simulink model "sim_req"  (R2021b)
settings: Solver=VariableStepAuto  StartTime=0.0  StopTime=10.0  RelTol=1e-3
settings Model: Creator=matas  LastModifiedBy=matas

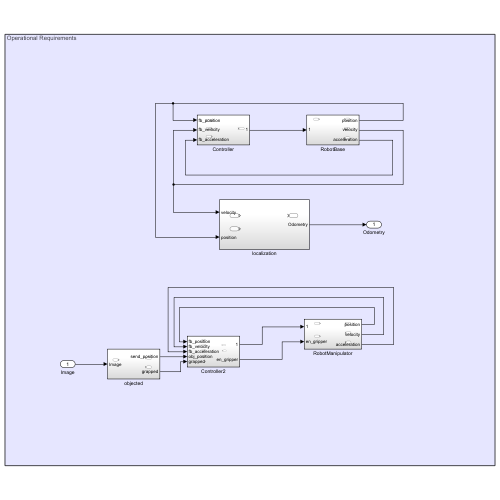
[thumbnail: Simulink's stored preview of the top-level diagram]
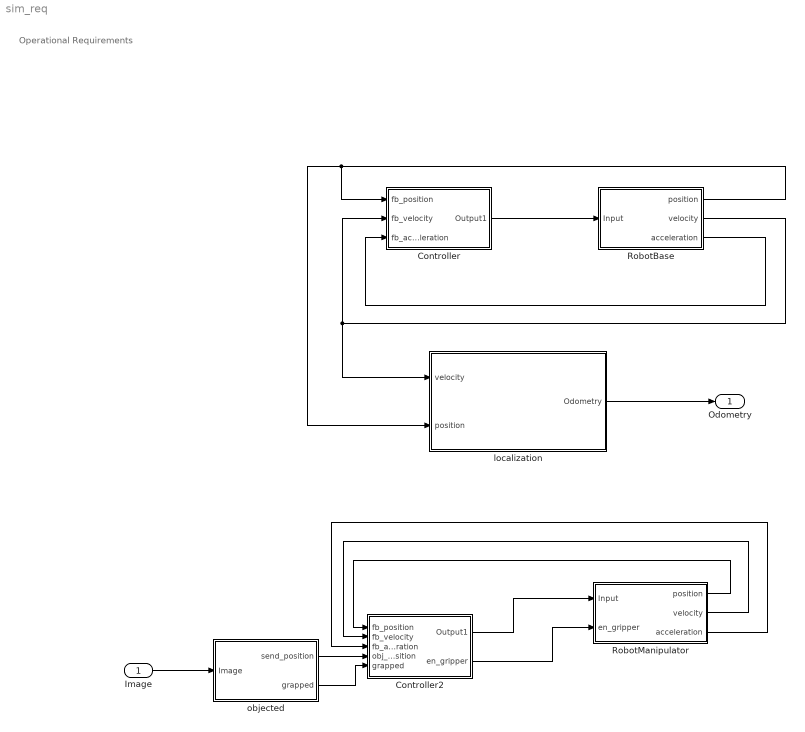
== system sim_req ==
  note: Operational Requirements
  Image : Inport
  Controller : Subsystem
  Controller2 : Subsystem
  RobotBase : Subsystem
  RobotManipulator : Subsystem
  localization : Subsystem
  objected : Subsystem
  Odometry : Outport
  wires:
  Controller/1(Output1) -> RobotBase/1(Input)
  RobotBase/1(position) -> Controller/1(fb_position), localization/2("position ")
  RobotBase/2(velocity) -> Controller/2(fb_velocity), localization/1(velocity)
  RobotBase/3(acceleration) -> Controller/3(fb_acceleration)
  localization/1(Odometry) -> Odometry/1
  RobotManipulator/1(position) -> Controller2/1(fb_position)
  RobotManipulator/2(velocity) -> Controller2/2(fb_velocity)
  RobotManipulator/3(acceleration) -> Controller2/3(fb_acceleration)
  Controller2/1(Output1) -> RobotManipulator/1(Input)
  Image/1 -> objected/1(Image)
  objected/1(send_position) -> Controller2/4(obj_position)
  Controller2/2(en_gripper) -> RobotManipulator/2(en_gripper)
  objected/2(grapped) -> Controller2/5(grapped)

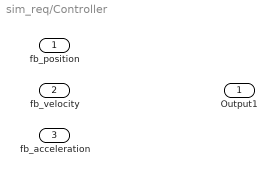
== system sim_req/Controller ==
  fb_position : Inport
  fb_velocity : Inport  Port=2
  fb_acceleration : Inport  Port=3
  Output1 : Outport

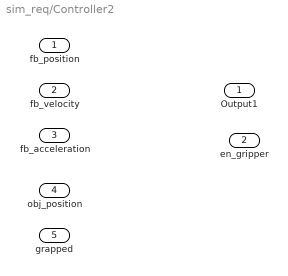
== system sim_req/Controller2 ==
  fb_position : Inport
  fb_velocity : Inport  Port=2
  fb_acceleration : Inport  Port=3
  obj_position : Inport  Port=4
  grapped : Inport  Port=5
  Output1 : Outport
  en_gripper : Outport  Port=2

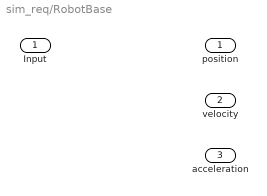
== system sim_req/RobotBase ==
  Input : Inport
  position : Outport
  velocity : Outport  Port=2
  acceleration : Outport  Port=3

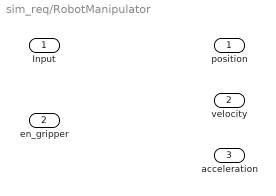
== system sim_req/RobotManipulator ==
  Input : Inport
  en_gripper : Inport  Port=2
  position : Outport
  velocity : Outport  Port=2
  acceleration : Outport  Port=3

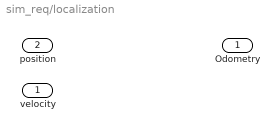
== system sim_req/localization ==
  velocity : Inport
  "position " : Inport  Port=2
  Odometry : Outport

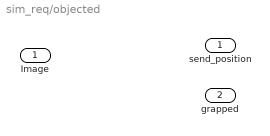
== system sim_req/objected ==
  Image : Inport
  send_position : Outport
  grapped : Outport  Port=2
